simulink model "parking"  (R2020b)
settings: Solver=VariableStepAuto  StartTime=0.0  StopTime=10  RelTol=1e-3
undefined symbols (not defined in the file or in its folder): car, car_LQR
libraries: fuzblock x1, simulink x1
settings Model: Creator=shima  LastModifiedBy=shima

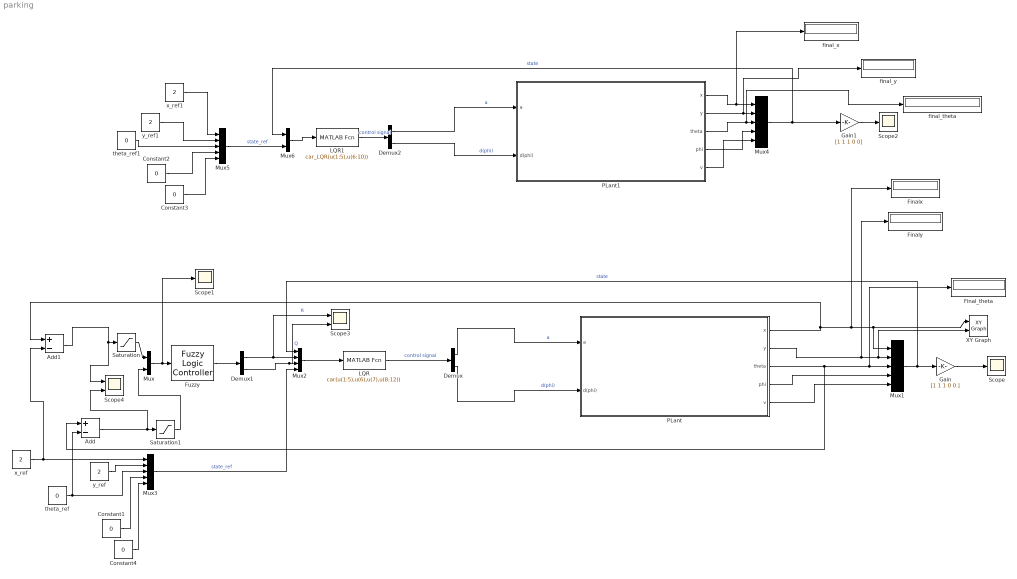
== system parking ==
  Add : Sum  Inputs=+-
  Add1 : Sum  Inputs=+-
  Constant{1..4} (4 alike) : Constant  Value=0
  Demux : Demux  Outputs=2
  Demux1 : Demux  Outputs=2
  Demux2 : Demux  Outputs=2
  Final_theta : Display
  Finalx : Display
  Finaly : Display
  Fuzzy : fuzblock/Fuzzy Logic  Controller  FIS='parking.fis'  OutputSampleNumber=101  DataType=double  FuzzifiedInputs=off  RuleFiringStrengths=off  RuleOutputs=off  AggregatedOutputs=off  SimulateUsing=Interpreted execution  OutOfRangeInputValueMessage=warning  NoRuleFiredMessage=warning  EmptyOutputFuzzySetMessage=warning
  Gain : Gain  Gain=[1 1 1 0 0 ]
  Gain1 : Gain  Gain=[1 1 1 0 0]
  LQR : MATLABFcn  MATLABFcn=car(u(1:5),u(6),u(7),u(8:12))  OutputDimensions=[2 1]  Output1D=off
  LQR1 : MATLABFcn  MATLABFcn=car_LQR(u(1:5),u(6:10))  OutputDimensions=[2 1]  Output1D=off
  Mux : Mux  Inputs=2
  Mux{1,3..5} (4 alike) : Mux  Inputs=5
  Mux2 : Mux
  Mux6 : Mux  Inputs=2
  PLant : Subsystem
  PLant1 : Subsystem
  Saturation : Saturate  UpperLimit=3  LowerLimit=-3  ZeroCross=off
  Saturation1 : Saturate  UpperLimit=pi/4  LowerLimit=-pi/4  ZeroCross=off
  Scope : Scope
  Scope1 : Scope
  Scope2 : Scope
  Scope3 : Scope  NumInputPorts=2
  Scope4 : Scope  NumInputPorts=2
  XY Graph : simulink/Sinks/XY Graph  xmin=-5  xmax=5  ymin=-5  ymax=5  st=-1
  final_theta : Display
  final_x : Display
  final_y : Display
  theta_ref : Constant  Value=0
  theta_ref1 : Constant  Value=0
  x_ref : Constant  Value=2
  x_ref1 : Constant  Value=2
  y_ref : Constant  Value=2
  y_ref1 : Constant  Value=2
  wires:
  PLant/3(theta) -> Add/1, Final_theta/1, Mux1/3
  Mux/1 -> Scope1/1, Fuzzy/1
  Demux/2 -> PLant/2(d(phi))  "d(phi)"
  Demux/1 -> PLant/1(a)  "a"
  Fuzzy/1 -> Demux1/1
  Demux1/1 -> Scope3/1, Mux2/2  "R"
  Demux1/2 -> Scope3/2, Mux2/3  "Q"
  Mux2/1 -> LQR/1
  x_ref/1 -> Add1/2, Mux3/1
  y_ref/1 -> Mux3/2
  Constant1/1 -> Mux3/4
  Constant4/1 -> Mux3/5
  PLant/1(x) -> Finalx/1, XY Graph/1, Mux1/1, Add1/1
  PLant/2(y) -> Finaly/1, XY Graph/2, Mux1/2
  PLant/4(phi) -> Mux1/4
  PLant/5(v) -> Mux1/5
  theta_ref/1 -> Add/2, Mux3/3
  Mux3/1 -> Mux2/4  "state_ref"
  Mux1/1 -> Gain/1, Mux2/1  "state"
  Gain/1 -> Scope/1
  LQR/1 -> Demux/1  "control signal"
  Saturation1/1 -> Mux/2
  PLant1/1(x) -> final_x/1, Mux4/1
  PLant1/2(y) -> final_y/1, Mux4/2
  PLant1/3(theta) -> final_theta/1, Mux4/3
  PLant1/4(phi) -> Mux4/4
  PLant1/5(v) -> Mux4/5
  LQR1/1 -> Demux2/1  "control signal"
  Demux2/1 -> PLant1/1(a)  "a"
  Demux2/2 -> PLant1/2(d(phi))  "d(phi)"
  Mux6/1 -> LQR1/1
  Mux4/1 -> Gain1/1, Mux6/1  "state"
  Mux5/1 -> Mux6/2  "state_ref"
  x_ref1/1 -> Mux5/1
  y_ref1/1 -> Mux5/2
  theta_ref1/1 -> Mux5/3
  Constant2/1 -> Mux5/4
  Constant3/1 -> Mux5/5
  Gain1/1 -> Scope2/1
  Add/1 -> Scope4/2, Saturation1/1
  Saturation/1 -> Mux/1
  Add1/1 -> Scope4/1, Saturation/1

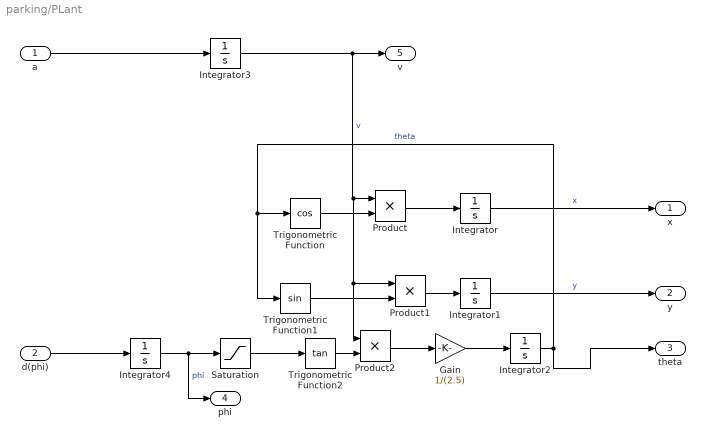
== system parking/PLant ==
  a : Inport
  d(phi) : Inport  Port=2
  Gain : Gain  Gain=1/(2.5)
  Integrator : Integrator
  Integrator1 : Integrator
  Integrator2 : Integrator  InitialCondition=.3
  Integrator3 : Integrator  InitialCondition=1
  Integrator4 : Integrator
  Product : Product
  Product1 : Product
  Product2 : Product
  Saturation : Saturate  UpperLimit=.52  LowerLimit=-0.52
  Trigonometric Function : Trigonometry  Operator=cos
  Trigonometric Function1 : Trigonometry
  Trigonometric Function2 : Trigonometry  Operator=tan
  x : Outport
  y : Outport  Port=2
  theta : Outport  Port=3
  phi : Outport  Port=4
  v : Outport  Port=5
  wires:
  Product/1 -> Integrator/1
  Trigonometric Function/1 -> Product/2
  Integrator2/1 -> theta/1, Trigonometric Function/1, Trigonometric Function1/1  "theta"
  Integrator4/1 -> phi/1, Saturation/1  "phi"
  Saturation/1 -> Trigonometric Function2/1
  Product2/1 -> Gain/1
  Trigonometric Function2/1 -> Product2/2
  Trigonometric Function1/1 -> Product1/2
  Gain/1 -> Integrator2/1
  Product1/1 -> Integrator1/1
  d(phi)/1 -> Integrator4/1
  a/1 -> Integrator3/1
  Integrator3/1 -> Product2/1, Product1/1, Product/1, v/1  "v"
  Integrator1/1 -> y/1  "y"
  Integrator/1 -> x/1  "x"

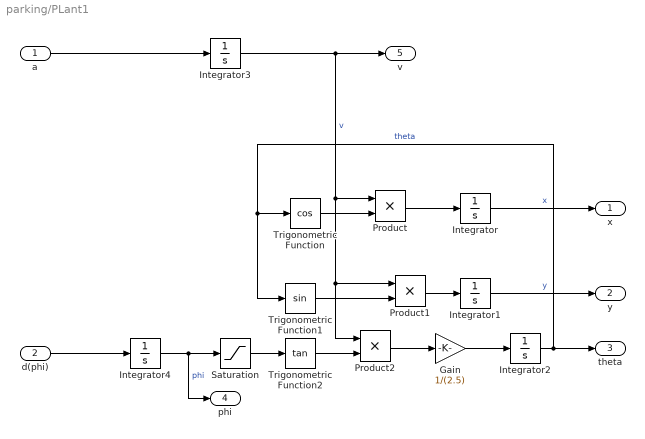
== system parking/PLant1 ==
  a : Inport
  d(phi) : Inport  Port=2
  Gain : Gain  Gain=1/(2.5)
  Integrator : Integrator
  Integrator1 : Integrator
  Integrator2 : Integrator  InitialCondition=.3
  Integrator3 : Integrator  InitialCondition=.5
  Integrator4 : Integrator
  Product : Product
  Product1 : Product
  Product2 : Product
  Saturation : Saturate  UpperLimit=.52  LowerLimit=-0.52
  Trigonometric Function : Trigonometry  Operator=cos
  Trigonometric Function1 : Trigonometry
  Trigonometric Function2 : Trigonometry  Operator=tan
  x : Outport
  y : Outport  Port=2
  theta : Outport  Port=3
  phi : Outport  Port=4
  v : Outport  Port=5
  wires:
  Product/1 -> Integrator/1
  Trigonometric Function/1 -> Product/2
  Integrator2/1 -> theta/1, Trigonometric Function/1, Trigonometric Function1/1  "theta"
  Integrator4/1 -> phi/1, Saturation/1  "phi"
  Saturation/1 -> Trigonometric Function2/1
  Product2/1 -> Gain/1
  Trigonometric Function2/1 -> Product2/2
  Trigonometric Function1/1 -> Product1/2
  Gain/1 -> Integrator2/1
  Product1/1 -> Integrator1/1
  d(phi)/1 -> Integrator4/1
  Integrator/1 -> x/1  "x"
  Integrator1/1 -> y/1  "y"
  a/1 -> Integrator3/1
  Integrator3/1 -> Product1/1, Product2/1, Product/1, v/1  "v"
